simulink model "test"  (R2020a)
settings: Solver=VariableStepAuto  StartTime=0.0  StopTime=30  RelTol=1e-3
model workspace (MAT data in the model file):
  Acc_command = Simulink.Parameter
  Acc_command.DataType = 'auto'
  Acc_command.Dimensions = [0 0]
  AngIn_command = Simulink.Parameter
  AngIn_command.DataType = 'auto'
  AngIn_command.Dimensions = [0 0]
  Dece_command = Simulink.Parameter
  Dece_command.DataType = 'auto'
  Dece_command.Dimensions = [0 0]
libraries: autolibutils x4, autolibshared x2, vehdynlibsteering x1, simulink x1, mpcadaslib x1
(part 1 of 3)
settings Model: PacingRate=1.100000  Creator=shiqihang  LastModifiedBy=qihan

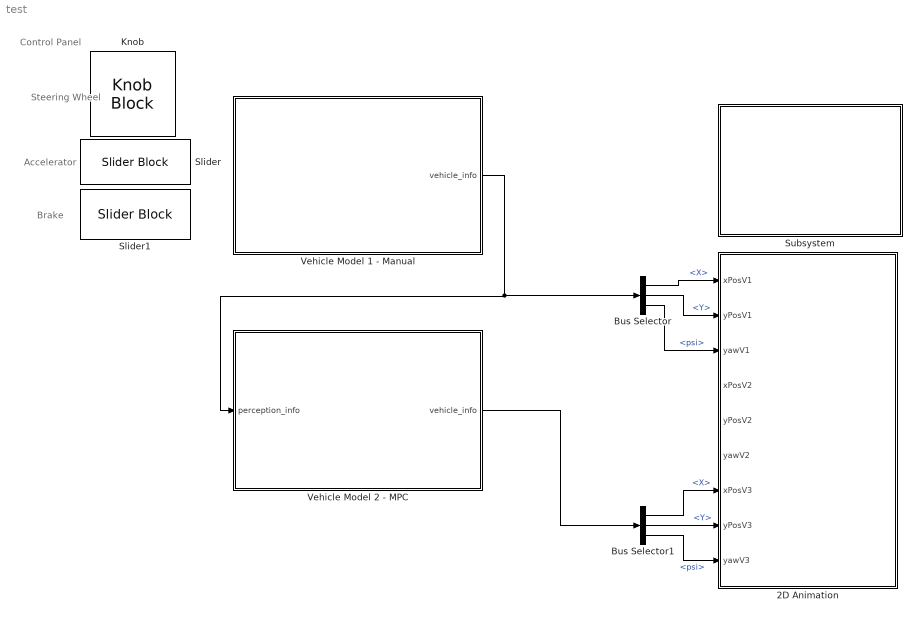
== system test ==
  note: Steering
      | Wheel
  note: Control Panel
  note: Accelerator
  note: Brake
  2D Animation : Subsystem  TreatAsAtomicUnit=on  SystemSampleTime=0.02
  Bus Selector : BusSelector  OutputSignals=InertFrm.Cg.Disp.X,InertFrm.Cg.Disp.Y,InertFrm.Cg.Ang.psi
  Bus Selector1 : BusSelector  OutputSignals=X,Y,psi
  Knob : KnobBlock  ScaleMin=-2  ScaleMax=2
  Slider : SliderBlock
  Slider1 : SliderBlock
  Subsystem : Subsystem
  Vehicle Model 1 - Manual : Subsystem  mask{X_init=50, xdot_init=10, Y_init=10, ydot_init=0, AngIn_command=-0.006511027018229143, Acc_command=0.3429878048780488, Dece_command=0}
      mask prompts: X_init "Initial X Position"; xdot_init "Initial Longitudinal Velocity"; Y_init "Initial Y Position"; ydot_init "Initial Lateral Velocity"; AngIn_command "Angle Command"; Acc_command "Acc Command"; Dece_command "Dece Command"
      mask Display: image('$imagefile'); % Use "Edit Image" on toolstrip to change.
  Vehicle Model 2 - MPC : Subsystem  mask{X_init=0, xdot_init=25, Y_init=0, ydot_init=0}
      mask prompts: X_init "Initial X Position"; xdot_init "Initial Longitudinal Velocity"; Y_init "Initial Y Position"; ydot_init "Initial Lateral Velocity"
      mask TypeOptions X_init: Initial Position Z/Value
      mask TypeOptions xdot_init: Initial Speed/Value
      mask Display: image('$imagefile'); % Use "Edit Image" on toolstrip to change.
  wires:
  Vehicle Model 1 - Manual/1(vehicle_info) -> Bus Selector/1, Vehicle Model 2 - MPC/1(perception_info)
  Bus Selector/1 -> 2D Animation/1(xPosV1)  "<X>"
  Bus Selector/2 -> 2D Animation/2(yPosV1)  "<Y>"
  Bus Selector/3 -> 2D Animation/3(yawV1)  "<psi>"
  Vehicle Model 2 - MPC/1(vehicle_info) -> Bus Selector1/1
  Bus Selector1/1 -> 2D Animation/7(xPosV3)  "<X>"
  Bus Selector1/2 -> 2D Animation/8(yPosV3)  "<Y>"
  Bus Selector1/3 -> 2D Animation/9(yawV3)  "<psi>"

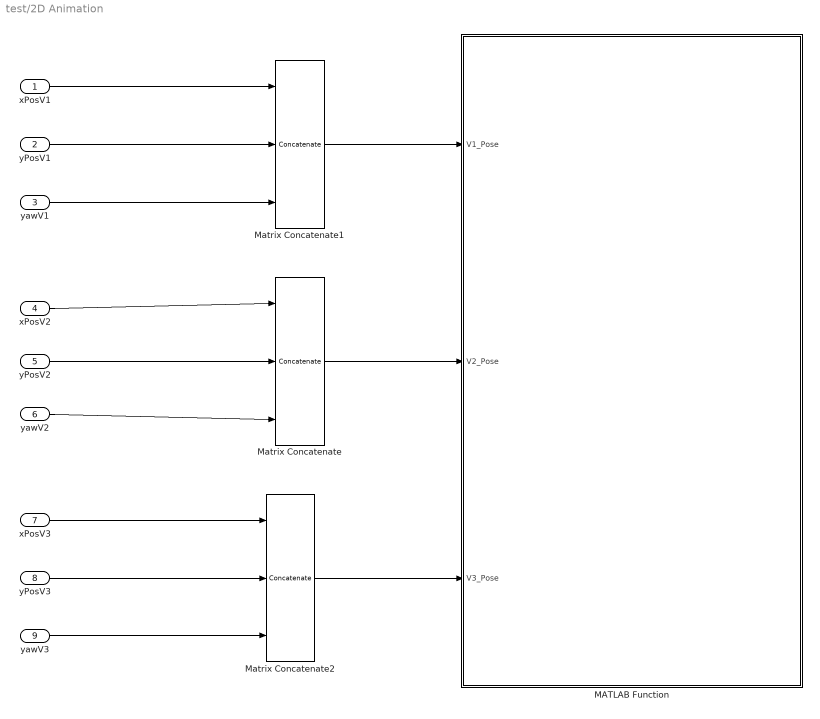
== system test/2D Animation ==
  xPosV1 : Inport
  yPosV1 : Inport  Port=2
  yawV1 : Inport  Port=3
  xPosV2 : Inport  Port=4
  yPosV2 : Inport  Port=5
  yawV2 : Inport  Port=6
  xPosV3 : Inport  Port=7
  yPosV3 : Inport  Port=8
  yawV3 : Inport  Port=9
  MATLAB Function : MATLAB Function  TreatAsAtomicUnit=on
      mask init:
      | close all;
      | figure('units','normalized','outerposition',[0 0 1 1]);
      | grid on
      | axis equal
      | hold on
  Matrix Concatenate : Concatenate  NumInputs=3  ConcatenateDimension=2
  Matrix Concatenate1 : Concatenate  NumInputs=3  ConcatenateDimension=2
  Matrix Concatenate2 : Concatenate  NumInputs=3  ConcatenateDimension=2
  wires:
  xPosV2/1 -> Matrix Concatenate/1
  Matrix Concatenate/1 -> MATLAB Function/2(V2_Pose)
  yPosV2/1 -> Matrix Concatenate/2
  yawV2/1 -> Matrix Concatenate/3
  Matrix Concatenate1/1 -> MATLAB Function/1(V1_Pose)
  xPosV1/1 -> Matrix Concatenate1/1
  yPosV1/1 -> Matrix Concatenate1/2
  yawV1/1 -> Matrix Concatenate1/3
  yPosV3/1 -> Matrix Concatenate2/2
  xPosV3/1 -> Matrix Concatenate2/1
  yawV3/1 -> Matrix Concatenate2/3
  Matrix Concatenate2/1 -> MATLAB Function/3(V3_Pose)

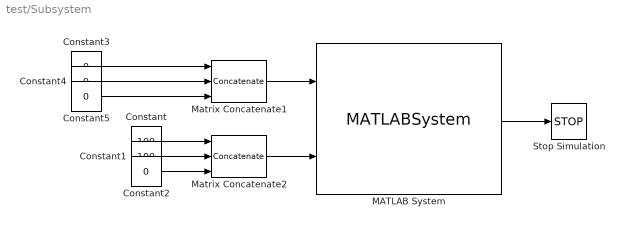
== system test/Subsystem ==
  Constant : Constant  Value=100
  Constant1 : Constant  Value=100
  Constant{2..5} (4 alike) : Constant  Value=0
  MATLAB System : MATLABSystem  System=collision_detection  v1_frame=[ 4, 2 ]  v2_frame=[ 4, 2 ]  SimulateUsing=Interpreted execution
      mask Type: collision_detection
      mask Display:
      | disp('collision_detection');
      | port_label('input',1,'v1_pos');
      | port_label('input',2,'v2_pos');
      | port_label('output',1,'collision_flag');
  Matrix Concatenate1 : Concatenate  NumInputs=3  Mode=Multidimensional array  ConcatenateDimension=2
  Matrix Concatenate2 : Concatenate  NumInputs=3  Mode=Multidimensional array  ConcatenateDimension=2
  Stop Simulation : Stop
  wires:
  MATLAB System/1 -> Stop Simulation/1
  Matrix Concatenate2/1 -> MATLAB System/2
  Matrix Concatenate1/1 -> MATLAB System/1
  Constant2/1 -> Matrix Concatenate2/3
  Constant1/1 -> Matrix Concatenate2/2
  Constant/1 -> Matrix Concatenate2/1
  Constant5/1 -> Matrix Concatenate1/3
  Constant4/1 -> Matrix Concatenate1/2
  Constant3/1 -> Matrix Concatenate1/1

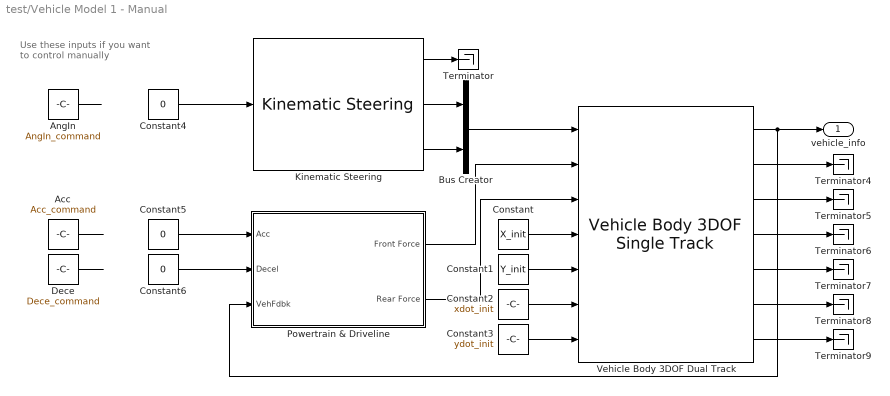
== system test/Vehicle Model 1 - Manual ==
  note: Use these inputs if
      | you want to control
      | manually
  Acc : Constant  Value=Acc_command
  AngIn : Constant  Value=AngIn_command
  Bus Creator : BusCreator  Inputs=2
  Constant : Constant  Value=X_init
  Constant1 : Constant  Value=Y_init
  Constant2 : Constant  Value=xdot_init
  Constant3 : Constant  Value=ydot_init
  Constant4 : Constant  Value=0
  Constant5 : Constant  Value=0
  Constant6 : Constant  Value=0
  Dece : Constant  Value=Dece_command
  Kinematic Steering : vehdynlibsteering/Kinematic Steering  StrgType=Rack and pinion  StrgRatioType=Constant  Loc=Front  NrmlFctr=0.01  TrckWdth=1  WhlBase=1.524  Db=0  StrgRng=1.25*pi  StrgAngBpts="[-6.2832   -5.0265   -3.7699   -2.5133   -1.2566         0    1.2566    2.5133    3.7699    5.0265    6.2832]"  StrgRatioTbl=|  StrgRatio=100  StrgArmLngth=0.1  RckCsLngth=0.5  TieRodLngth=0.248  D=0.2  PnnRadius=0.0057  PnnRadiusTbl="[0.0055    0.0055    0.0056    0.0057    0.0058    0.0057    0.0057    0.0057    0.0056    0.0055    0.0055]"  RodLngth=0.1  ParaArmLngth=0.9  aMode=2
      | [13.5000   13.3750   13.2500   13.1250   13.0000   13.0000   13.0000   13.1250   13.2500   13.3750   13.5000
      | ]
  Powertrain & Driveline : Subsystem
      mask Display: image('vdbslibpt.png');
  Terminator{,4..9} (7 alike) : Terminator
  Vehicle Body 3DOF Dual Track : autolibshared/Vehicle Body 3DOF Single Track  trackMode=Dual  inputMode=External longitudinal forces  frontSteerMode=on  rearSteerMode=off  windMode=off  muMode=off  extFMode=off  extMMode=off  extXo=on  extpsio=off  extxdoto=on  extro=off  extYo=on  extTamb=off  extydoto=on  aMode=2  NF=2  NR=2  m=2000  a=1.4  b=1.6  h=0.35  X_o=0  xdot_o=0  CalphaMode=off  sigmaMode=on  d=0  w=[1.4,1.4]  Cy_f=12e3  Cy_r=11e3  sigma_f=.1  sigma_r=.1  alpha_f_brk=[-.1 .1]  Cy_f_data=[-9e3 9e3]  alpha_r_brk=[-.1 .1]  Cy_r_data=[-9e3 9e3]  Y_o=0  ydot_o=0  Izz=4000  psi_o=0  r_o=0  Af=2  Cd=.3  Cl=.1  Cpm=.1  beta_w=[0:0.01:0.3]  Cs=[0:0.03:0.9]  Cym=[0:0.01:0.3]  Pabs=101325  Tair=273  g=9.81  mu=1  xdot_tol=.01  Fznom=5000  Fxtire_sat=7e4  Fytire_sat=7e4  longOff=0  latOff=0  vertOff=0  wrapAng=off
      settings: SourceProductBaseCode=PW,MT,VE,VP
  vehicle_info : Outport
  wires:
  Dece/1 -> ?
  AngIn/1 -> ?
  Kinematic Steering/3 -> Bus Creator/2
  Vehicle Body 3DOF Dual Track/4 -> Terminator6/1
  Acc/1 -> ?
  Vehicle Body 3DOF Dual Track/2 -> Terminator4/1
  Vehicle Body 3DOF Dual Track/6 -> Terminator8/1
  Powertrain & Driveline/2(Rear Force) -> Vehicle Body 3DOF Dual Track/3
  Vehicle Body 3DOF Dual Track/1 -> Powertrain & Driveline/3(VehFdbk), vehicle_info/1
  Vehicle Body 3DOF Dual Track/5 -> Terminator7/1
  Powertrain & Driveline/1(Front Force) -> Vehicle Body 3DOF Dual Track/2
  Kinematic Steering/1 -> Terminator/1
  Vehicle Body 3DOF Dual Track/3 -> Terminator5/1
  Bus Creator/1 -> Vehicle Body 3DOF Dual Track/1
  Vehicle Body 3DOF Dual Track/7 -> Terminator9/1
  Kinematic Steering/2 -> Bus Creator/1
  Constant3/1 -> Vehicle Body 3DOF Dual Track/7
  Constant2/1 -> Vehicle Body 3DOF Dual Track/6
  Constant1/1 -> Vehicle Body 3DOF Dual Track/5
  Constant/1 -> Vehicle Body 3DOF Dual Track/4
  Constant4/1 -> Kinematic Steering/1
  Constant6/1 -> Powertrain & Driveline/2(Decel)
  Constant5/1 -> Powertrain & Driveline/1(Acc)

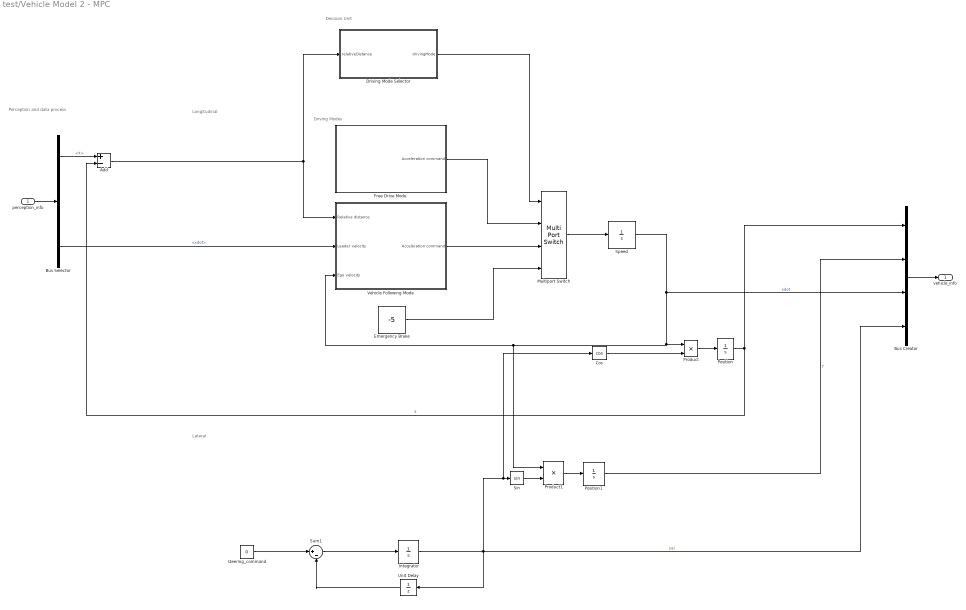
== system test/Vehicle Model 2 - MPC ==
  note: Perception and data process
  note: Lateral
  note: Longitudinal
  note: Driving Modes
  note: Decision Unit
  perception_info : Inport
  Add : Sum  Inputs=+-
  Bus Creator : BusCreator  Inputs=4
  Bus Selector : BusSelector  OutputSignals=InertFrm.Cg.Disp.X,InertFrm.Cg.Disp.Y,BdyFrm.Cg.Vel.xdot
  Cos : Trigonometry  Operator=cos
  Driving Mode Selector : Stateflow chart  TreatAsAtomicUnit=on
  Emergency Brake : Constant  Value=-5
  Free Drive Mode : Subsystem
  Integrator : Integrator
  Multiport Switch : MultiPortSwitch
  Position : Integrator  InitialCondition=X_init
  Position1 : Integrator  InitialCondition=Y_init
  Product : Product
  Product1 : Product
  Sin : Trigonometry
  Speed : Integrator  InitialCondition=xdot_init  LimitOutput=on  LowerSaturationLimit=0
  Sum1 : Sum  Inputs=|+-
  Unit Delay : UnitDelay  SampleTime=-1  HasFrameUpgradeWarning=on
  Vehicle Following Mode : Subsystem
  steering_command : Constant  Value=0
  vehicle_info : Outport
  wires:
  Driving Mode Selector/1(drivingMode) -> Multiport Switch/1
  Emergency Brake/1 -> Multiport Switch/4
  Free Drive Mode/1(Acceleration command) -> Multiport Switch/2
  Multiport Switch/1 -> Speed/1
  Vehicle Following Mode/1(Acceleration command) -> Multiport Switch/3
  Bus Selector/3 -> Vehicle Following Mode/2(Leader velocity)  "<xdot>"
  Add/1 -> Vehicle Following Mode/1(Relative distance), Driving Mode Selector/1(relativeDistance)
  Position1/1 -> Bus Creator/2  "Y"
  Product1/1 -> Position1/1
  Sin/1 -> Product1/2
  Product/1 -> Position/1
  Cos/1 -> Product/2
  Unit Delay/1 -> Sum1/2
  Integrator/1 -> Bus Creator/4, Cos/1, Sin/1, Unit Delay/1  "psi"
  Sum1/1 -> Integrator/1
  steering_command/1 -> Sum1/1
  Speed/1 -> Product1/1, Vehicle Following Mode/3(Ego velocity), Product/1, Bus Creator/3  "xdot"
  Position/1 -> Bus Creator/1, Add/2  "X"
  perception_info/1 -> Bus Selector/1
  Bus Selector/1 -> Add/1  "<X>"
  Bus Creator/1 -> vehicle_info/1

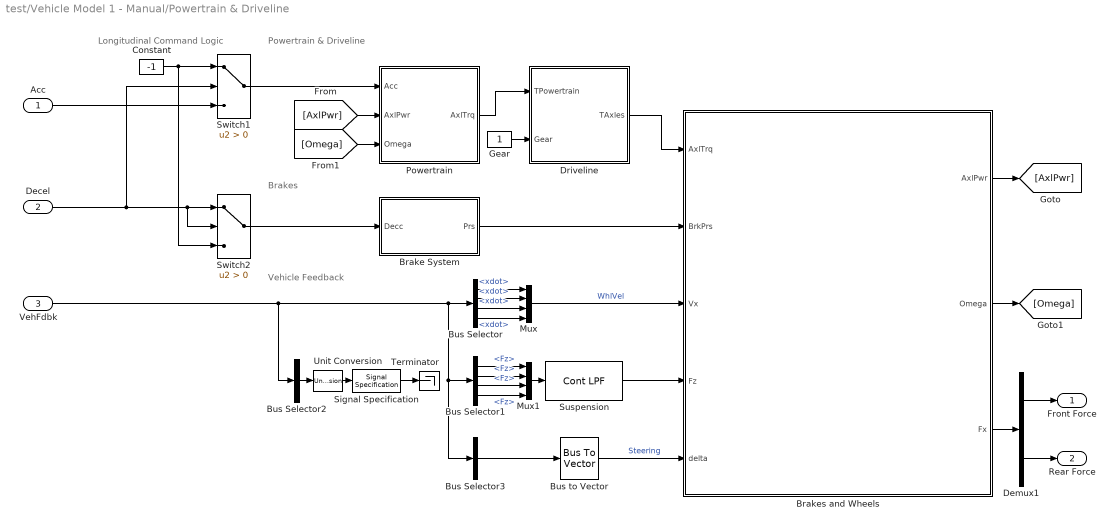
== system test/Vehicle Model 1 - Manual/Powertrain & Driveline ==
  note: Longitudinal Command Logic
  note: Brakes
  note: Powertrain & Driveline
  note: Vehicle Feedback
  Acc : Inport
  Decel : Inport  Port=2
  VehFdbk : Inport  Port=3
  Brake System : Subsystem
  Brakes and Wheels : Subsystem  TreatAsAtomicUnit=on
      mask Display: image('vdbslibwhls.png');
  Bus Selector : BusSelector  OutputSignals=BdyFrm.FrntAxl.Lft.Vel.xdot,BdyFrm.FrntAxl.Rght.Vel.xdot,BdyFrm.RearAxl.Lft.Vel.xdot,BdyFrm.RearAxl.Rght.Vel.xdot
  Bus Selector1 : BusSelector  OutputSignals=BdyFrm.Forces.FrntAxl.Lft.Fz,BdyFrm.Forces.FrntAxl.Rght.Fz,BdyFrm.Forces.RearAxl.Lft.Fz,BdyFrm.Forces.RearAxl.Rght.Fz
  Bus Selector2 : BusSelector  OutputSignals=BdyFrm.Cg.Vel.xdot  OutputAsBus=on
  Bus Selector3 : BusSelector  OutputSignals=BdyFrm.FrntAxl.Steer.WhlAngFL,BdyFrm.FrntAxl.Steer.WhlAngFR,BdyFrm.RearAxl.Steer.WhlAngRL,BdyFrm.RearAxl.Steer.WhlAngRR  OutputAsBus=on
  Bus to Vector : BusToVector
  Constant : Constant  Value=-1
  Demux1 : Demux  Outputs=[2 2]
  Driveline : Subsystem  Variant=on  VariantControlMode=Label  VariantControl=Variant1  LabelModeActiveChoice=0
  Gear : Constant
  Mux : Mux
  Mux1 : Mux
  Powertrain : Subsystem
  Signal Specification : SignalSpecification  Unit=km/hr
  Suspension : autolibutils/Cont LPF  wc=10*pi*2  aMode=2
      settings: SourceProductBaseCode=PW,MT,VE,VP
  Switch1 : Switch  Criteria=u2 > Threshold
  Switch2 : Switch  Criteria=u2 > Threshold
  Terminator : Terminator
  Unit Conversion : UnitConversion
  Front Force : Outport  VectorParamsAs1DForOutWhenUnconnected=off
  Rear Force : Outport  Port=2  VectorParamsAs1DForOutWhenUnconnected=off
  wires:
  Decel/1 -> Switch1/2, Switch2/2, Switch2/1
  Acc/1 -> Switch1/3
  Constant/1 -> Switch2/3, Switch1/1
  Mux/1 -> Brakes and Wheels/3(Vx)  "WhlVel"
  VehFdbk/1 -> Bus Selector2/1, Bus Selector3/1, Bus Selector1/1, Bus Selector/1
  Demux1/1 -> Front Force/1
  Demux1/2 -> Rear Force/1
  Driveline/1(TAxles) -> Brakes and Wheels/1(AxlTrq)
  Brakes and Wheels/1(AxlPwr) -> [AxlPwr]
  Brakes and Wheels/3(Fx) -> Demux1/1
  Bus Selector3/1 -> Bus to Vector/1
  Bus to Vector/1 -> Brakes and Wheels/5(delta)  "Steering"
  Mux1/1 -> Suspension/1
  Suspension/1 -> Brakes and Wheels/4(Fz)
  Bus Selector/1 -> Mux/1  "<xdot>"
  Bus Selector/2 -> Mux/2  "<xdot>"
  Bus Selector/3 -> Mux/3  "<xdot>"
  Bus Selector/4 -> Mux/4  "<xdot>"
  Bus Selector1/1 -> Mux1/1  "<Fz>"
  Bus Selector1/2 -> Mux1/2  "<Fz>"
  Bus Selector1/3 -> Mux1/3  "<Fz>"
  Bus Selector1/4 -> Mux1/4  "<Fz>"
  Switch1/1 -> Powertrain/1(Acc)
  Powertrain/1(AxlTrq) -> Driveline/1(TPowertrain)
  Brakes and Wheels/2(Omega) -> [Omega]
  [AxlPwr] -> Powertrain/2(AxlPwr)
  [Omega] -> Powertrain/3(Omega)
  Switch2/1 -> Brake System/1(Decc)
  Brake System/1(Prs) -> Brakes and Wheels/2(BrkPrs)
  Bus Selector2/1 -> Unit Conversion/1
  Unit Conversion/1 -> Signal Specification/1
  Signal Specification/1 -> Terminator/1
  Gear/1 -> Driveline/2(Gear)

== system test/Vehicle Model 2 - MPC/Free Drive Mode ==
  Acc Command : Saturate  UpperLimit=2  LowerLimit=-3
  Acc Dynamics : TransferFcn  Denominator=[0.5 1]
  Constant : Constant  Value=xdot_init
  Sum13 : Sum  Inputs=|+-
  Acceleration command : Outport
  wires:
  Acc Command/1 -> Acc Dynamics/1
  Constant/1 -> Sum13/1
  Acc Dynamics/1 -> Sum13/2, Acceleration command/1
  Sum13/1 -> Acc Command/1

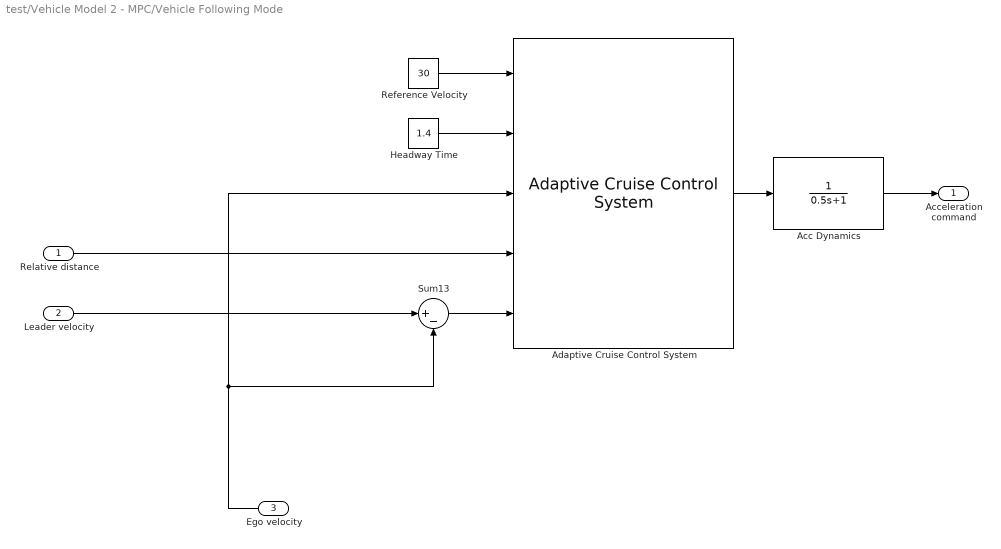
== system test/Vehicle Model 2 - MPC/Vehicle Following Mode ==
  Relative distance : Inport
  Leader velocity : Inport  Port=2
  Ego velocity : Inport  Port=3
  Acc Dynamics : TransferFcn  Denominator=[0.5 1]
  Adaptive Cruise Control System : mpcadaslib/Adaptive Cruise Control System  EgoModel=tf(1,[0.5,1,0])  InitialEgoVelocity=30  DefaultSpacing=10  MaxVelocity=50  MinAcceleration=-3  amin_ext=off  MaxAcceleration=2  amax_ext=off  Ts=0.5  PredictionHorizon=200  ControllerBehavior=0.590  suboptimal=off  maxiter=100  datatypeopt=double  optmode=off  trackmode=off
  Headway Time : Constant  Value=1.4
  Reference Velocity : Constant  Value=30
  Sum13 : Sum  Inputs=|+-
  Acceleration command : Outport
  wires:
  Acc Dynamics/1 -> Acceleration command/1
  Adaptive Cruise Control System/1 -> Acc Dynamics/1
  Relative distance/1 -> Adaptive Cruise Control System/4
  Sum13/1 -> Adaptive Cruise Control System/5
  Ego velocity/1 -> Sum13/2, Adaptive Cruise Control System/3
  Reference Velocity/1 -> Adaptive Cruise Control System/1
  Headway Time/1 -> Adaptive Cruise Control System/2
  Leader velocity/1 -> Sum13/1

== system test/Vehicle Model 1 - Manual/Powertrain & Driveline/Brake System ==
  Decc : Inport
  Hydraulics : autolibutils/Cont LPF  wc=30*pi*2  aMode=2
      settings: SourceProductBaseCode=PW,MT,VE,VP
  Pressure : Gain  Gain=2e7
  Saturation1 : Saturate  UpperLimit=inf  LowerLimit=0  ZeroCross=off
  Selector : Selector  InputPortWidth=1  IndexOptions=Index vector (dialog)  Indices=[1 1 1 1]  OutputSizes=1
  Signal Specification : SignalSpecification  Unit=Pa
  Prs : Outport  VectorParamsAs1DForOutWhenUnconnected=off
  wires:
  Pressure/1 -> Selector/1
  Hydraulics/1 -> Pressure/1
  Saturation1/1 -> Hydraulics/1
  Selector/1 -> Signal Specification/1
  Decc/1 -> Saturation1/1
  Signal Specification/1 -> Prs/1
